simulink model "simulink状态方程建模"  (R2021a)
settings: Solver=FixedStepAuto  StartTime=0.0  StopTime=20.0  FixedStep=0.1  RelTol=1e-3
settings Model: Creator=86137  LastModifiedBy=86137

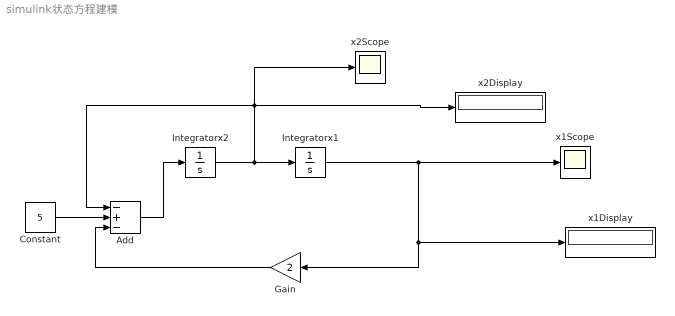
== system simulink状态方程建模 ==
  Add : Sum  Inputs=-+-
  Constant : Constant  Value=5
  Gain : Gain  Gain=2
  Integratorx1 : Integrator
  Integratorx2 : Integrator  InitialCondition=1
  x1Display : Display
  x1Scope : Scope
  x2Display : Display
  x2Scope : Scope
  wires:
  Integratorx1/1 -> Gain/1, x1Display/1, x1Scope/1
  Gain/1 -> Add/3
  Constant/1 -> Add/2
  Add/1 -> Integratorx2/1
  Integratorx2/1 -> x2Display/1, x2Scope/1, Add/1, Integratorx1/1
